simulink model "PID_Control"  (R2024a)
settings: Solver=FixedStepDiscrete  StartTime=0.0  StopTime=inf  FixedStep=0.001  RelTol=1e-3
libraries: simulink x5, arduinolib x3, arduinosensorlib x1
settings Model: ExtModeTrigDuration=2  Creator=lenovo  LastModifiedBy=lenovo
settings SolverCC: AutoInsertRateTranBlk=on
settings OptimizationCC: EnhancedBackFolding=on  PassReuseOutputArgsAs=Individual arguments  ZeroExternalMemoryAtStartup=off  ZeroInternalMemoryAtStartup=off  MaxStackSize=64  OptimizeBlockOrder=speed  DifferentSizesBufferReuse=on  OptimizationCustomize=off  EfficientTunableParamExpr=on
settings DebuggingCC: ParameterTunabilityLossMsg=error
settings HardwareCC: ProdBitPerInt=16  ProdBitPerPointer=16  ProdBitPerSizeT=16  ProdBitPerPtrDiffT=16  ProdLargestAtomicFloat=None  ProdWordSize=8  ProdHWDeviceType=Atmel->AVR
settings SFSimCC: MATLABDynamicMemAlloc=off
settings RTWCC: Description=Embedded Coder  SystemTargetFile=ert.tlc  HardwareBoard=Arduino Mega 2560  TemplateMakefile=ert_default_tmf  Toolchain=Arduino AVR
settings CodeAppCC: ForceParamTrailComments=on  IgnoreCustomStorageClasses=off  OperatorAnnotations=on  SimulinkDataObjDesc=on  SFDataObjDesc=on  InsertBlockDesc=on
settings ERTTargetCC: SupportContinuousTime=on  SupportVariableSizeSignals=on  ExtModeTransport=3  ExtModeStaticAlloc=on  ExtModeAutomaticAllocSize=off  ExtModeStaticAllocSize=2048  ExtModeMexFile=ext_xcp  ExtModeIntrfLevel=Level2 - Open

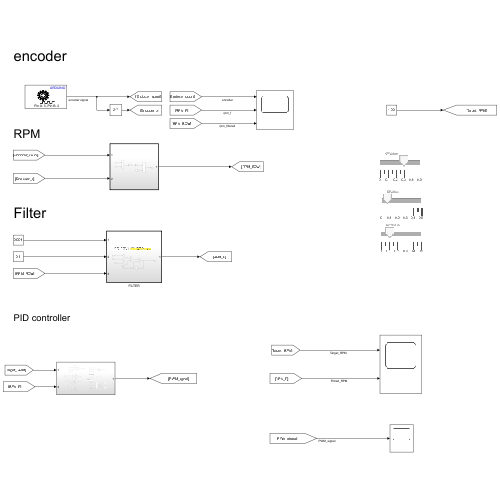
[thumbnail: Simulink's stored preview of the top-level diagram]
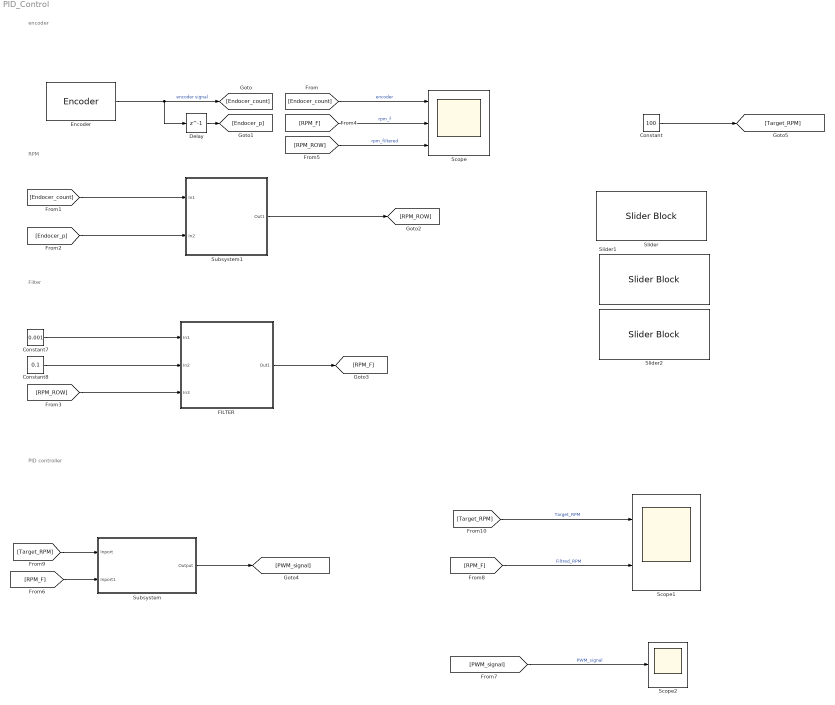
== system PID_Control ==
  note: PID controller
  note: RPM
  note: encoder
  note: Filter
  Constant : Constant  Value=100
  Constant7 : Constant  Value=0.001
  Constant8 : Constant  Value=0.1
  Delay : Delay  DelayLength=1
  Encoder : arduinosensorlib/Encoder  InputA=3  InputB=2  Mode=No reset  SampleTime=-1
  FILTER : Subsystem  TreatAsAtomicUnit=on
  Scope : Scope  NumInputPorts=3
  Scope1 : Scope  NumInputPorts=2
  Scope2 : Scope
  Slider : SliderBlock  ScaleMax=0.5
  Slider1 : SliderBlock  ScaleMax=0.5
  Slider2 : SliderBlock  ScaleMax=0.5
  Subsystem : Subsystem
  Subsystem1 : Subsystem  TreatAsAtomicUnit=on
  wires:
  Encoder/1 -> [Endocer_count], Delay/1  "encoder signal"
  [Endocer_count] -> Scope/1  "encoder"
  Delay/1 -> [Endocer_p]
  [RPM_F] -> Scope/2  "rpm_f"
  [RPM_ROW] -> Scope/3  "rpm_filtered"
  [Endocer_count] -> Subsystem1/1(In1)
  [Endocer_p] -> Subsystem1/2(In2)
  Subsystem1/1(Out1) -> [RPM_ROW]
  Constant7/1 -> FILTER/1(In1)
  [RPM_ROW] -> FILTER/3(In3)
  FILTER/1(Out1) -> [RPM_F]
  Constant8/1 -> FILTER/2(In2)
  [Target_RPM] -> Subsystem/1(Inport)
  [RPM_F] -> Subsystem/2(Inport1)
  Subsystem/1(Output) -> [PWM_signal]
  [RPM_F] -> Scope1/2  "Filtred_RPM"
  Constant/1 -> [Target_RPM]
  [Target_RPM] -> Scope1/1  "Target_RPM"
  [PWM_signal] -> Scope2/1  "PWM_signal"

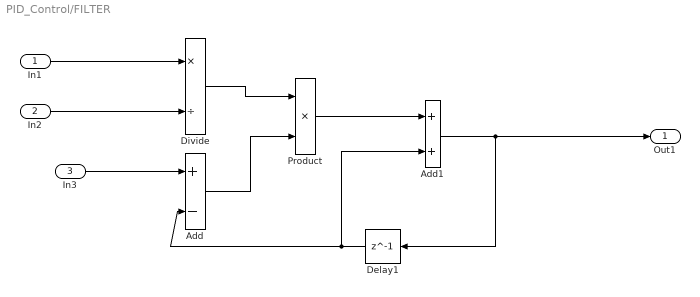
== system PID_Control/FILTER ==
  In1 : Inport
  In2 : Inport  Port=2
  In3 : Inport  Port=3
  Add : Sum  Inputs=+-
  Add1 : Sum
  Delay1 : Delay  DelayLength=1
  Divide : Product  Inputs=*/
  Product : Product
  Out1 : Outport
  wires:
  Add1/1 -> Out1/1, Delay1/1
  Divide/1 -> Product/1
  In2/1 -> Divide/2
  Delay1/1 -> Add1/2, Add/2
  Product/1 -> Add1/1
  In3/1 -> Add/1
  Add/1 -> Product/2
  In1/1 -> Divide/1

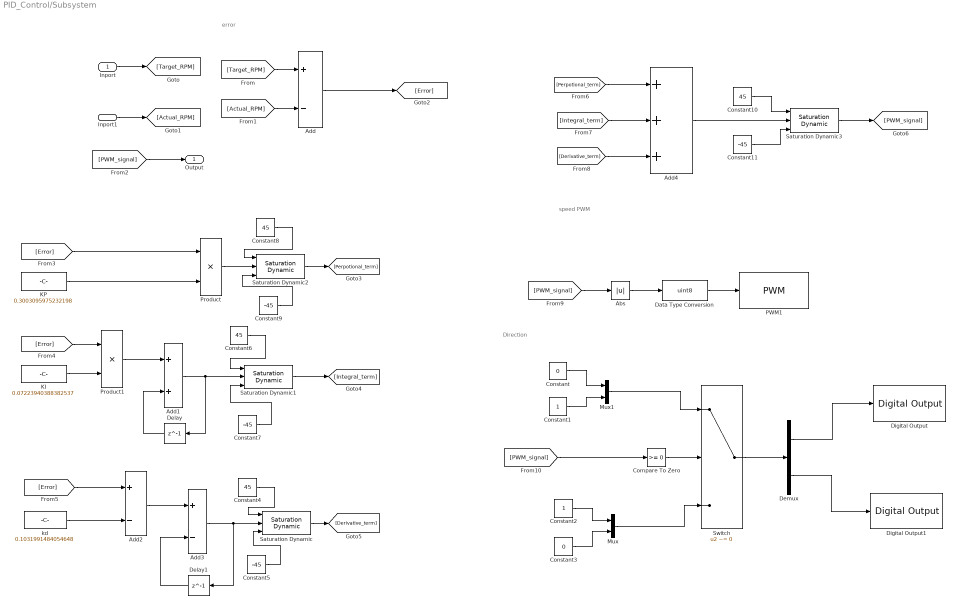
== system PID_Control/Subsystem ==
  note: error
  note: speed PWM
  note: Direction
  Inport : Inport
  Inport1 : Inport  Port=2
  Abs : Abs  SaturateOnIntegerOverflow=off
  Add : Sum  Inputs=+-
  Add1 : Sum
  Add2 : Sum  Inputs=+-
  Add3 : Sum  Inputs=+-
  Add4 : Sum  Inputs=+++
  Compare To Zero : simulink/Logic and Bit Operations/Compare To Zero  relop=>=  OutDataTypeStr=boolean
  Constant : Constant  Value=0
  Constant1 : Constant
  Constant{4,6,8,10} (4 alike) : Constant  Value=45
  Constant{5,7,9,11} (4 alike) : Constant  Value=-45
  Constant2 : Constant
  Constant3 : Constant  Value=0
  Data Type Conversion : DataTypeConversion  OutMin=0  OutMax=255  OutDataTypeStr=uint8  SaturateOnIntegerOverflow=off  RndMeth=Floor
  Delay : Delay  DelayLength=1
  Delay1 : Delay  DelayLength=1
  Demux : Demux  Outputs=2
  Digital Output : arduinolib/Digital Output  pinNumber=5  Direction=output  blockPlatform=arduino
  Digital Output1 : arduinolib/Digital Output  pinNumber=6  Direction=output  blockPlatform=arduino
  KI : Constant  Value=0.07223940388382537
  KP : Constant  Value=0.3003095975232198
  Mux : Mux  Inputs=2
  Mux1 : Mux  Inputs=2
  PWM1 : arduinolib/PWM  pinNumber=7  frequencyType=Default  desiredFrequency=490.2  achievableFrequency=490.2
  Product : Product
  Product1 : Product
  Saturation Dynamic{,1..3} (4 alike) : simulink/Discontinuities/Saturation Dynamic  OutMin=[]  OutMax=[]  OutDataTypeStr=Inherit: Same as second input  OutDataType=fixdt(1, 16)  OutScaling=2^-10  DoSatur=off
  Switch : Switch  Criteria=u2 ~= 0  SaturateOnIntegerOverflow=off  InputSameDT=off
  kd : Constant  Value=0.1031991484054648
  Output : Outport
  wires:
  Inport/1 -> [Target_RPM]
  Inport1/1 -> [Actual_RPM]
  [PWM_signal] -> Output/1
  [Target_RPM] -> Add/1
  [Actual_RPM] -> Add/2
  Add/1 -> [Error]
  [Error] -> Product/1
  KP/1 -> Product/2
  KI/1 -> Product1/2
  [Error] -> Product1/1
  Product1/1 -> Add1/1
  Add1/1 -> Saturation Dynamic1/2, Delay/1
  Delay/1 -> Add1/2
  [Error] -> Add2/1
  kd/1 -> Add2/2
  Add2/1 -> Add3/1
  Delay1/1 -> Add3/2
  Add3/1 -> Saturation Dynamic/2, Delay1/1
  [Integral_term] -> Add4/2
  [Perpotional_term] -> Add4/1
  [Derivative_term] -> Add4/3
  Data Type Conversion/1 -> PWM1/1
  [PWM_signal] -> Abs/1
  Mux1/1 -> Switch/1
  Demux/1 -> Digital Output/1
  Constant1/1 -> Mux1/2
  Constant/1 -> Mux1/1
  Constant3/1 -> Mux/2
  Mux/1 -> Switch/3
  Constant2/1 -> Mux/1
  Demux/2 -> Digital Output1/1
  Switch/1 -> Demux/1
  [PWM_signal] -> Compare To Zero/1
  Abs/1 -> Data Type Conversion/1
  Compare To Zero/1 -> Switch/2
  Constant4/1 -> Saturation Dynamic/1
  Constant5/1 -> Saturation Dynamic/3
  Saturation Dynamic/1 -> [Derivative_term]
  Constant6/1 -> Saturation Dynamic1/1
  Constant7/1 -> Saturation Dynamic1/3
  Saturation Dynamic1/1 -> [Integral_term]
  Constant8/1 -> Saturation Dynamic2/1
  Constant9/1 -> Saturation Dynamic2/3
  Saturation Dynamic2/1 -> [Perpotional_term]
  Product/1 -> Saturation Dynamic2/2
  Constant10/1 -> Saturation Dynamic3/1
  Constant11/1 -> Saturation Dynamic3/3
  Saturation Dynamic3/1 -> [PWM_signal]
  Add4/1 -> Saturation Dynamic3/2

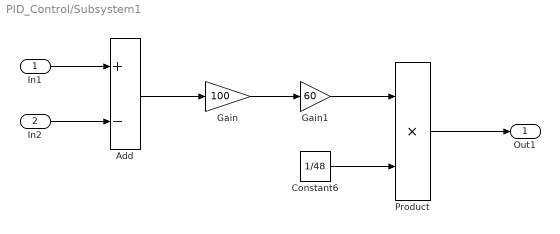
== system PID_Control/Subsystem1 ==
  In1 : Inport
  In2 : Inport  Port=2
  Add : Sum  Inputs=+-
  Constant6 : Constant  Value=1/48
  Gain : Gain  Gain=100
  Gain1 : Gain  Gain=60
  Product : Product
  Out1 : Outport
  wires:
  Constant6/1 -> Product/2
  Gain/1 -> Gain1/1
  In2/1 -> Add/2
  Add/1 -> Gain/1
  Gain1/1 -> Product/1
  Product/1 -> Out1/1
  In1/1 -> Add/1
